simulink model "EspacioDeEstados"  (Simulink 7.9)
settings: Solver=ode45  StartTime=0.0  StopTime=50.0  RelTol=1e-3
undefined symbols (not defined in the file or in its folder): A, B
settings Model: Creator=Paul  LastModifiedBy=Santiago
settings DataIOCC: SignalLoggingSaveFormat=Dataset
settings OptimizationCC: ExpressionDepthLimit=128
settings DebuggingCC: MultiTaskDSMMsg=warning  MultiTaskCondExecSysMsg=none  StrictBusMsg=None
settings RTWCC: IncludeERTFirstTime=on
settings CodeAppCC: CustomSymbolStrType=$N$R$M_T

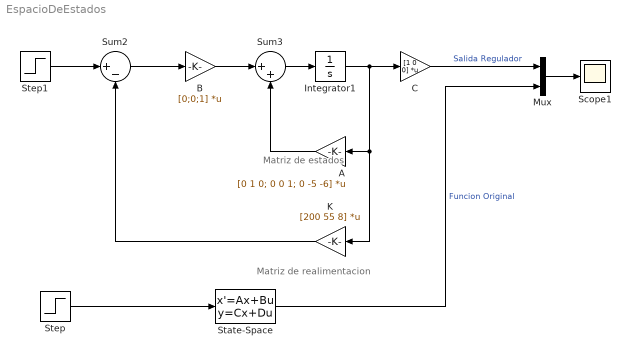
== system EspacioDeEstados ==
  note: Matriz de realimentacion
  note: Matriz de estados
  A : Gain  Gain=[0 1 0; 0 0 1; 0 -5 -6]  Multiplication=Matrix(K*u)
  B : Gain  Gain=[0;0;1]  Multiplication=Matrix(K*u)
  C : Gain  Gain=[1 0 0]  Multiplication=Matrix(K*u)
  Integrator1 : Integrator  InitialCondition=1
  K : Gain  Gain=[200 55 8]  Multiplication=Matrix(K*u)
  Mux : Mux  Inputs=2
  Scope1 : Scope
      settings: ShowLegends=on
  State-Space : StateSpace  A=A  B=B  C=[1 0 0]  D=0  X0=[1 1 1]
  Step : Step  After=0  SampleTime=0
  Step1 : Step  Time=0  After=0  SampleTime=0
  Sum2 : Sum  Inputs=|+-
  Sum3 : Sum  Inputs=|++
  wires:
  Step1/1 -> Sum2/1
  Sum2/1 -> B/1
  B/1 -> Sum3/1
  Sum3/1 -> Integrator1/1
  A/1 -> Sum3/2
  K/1 -> Sum2/2
  Integrator1/1 -> K/1, A/1, C/1
  C/1 -> Mux/1  "Salida Regulador"
  Mux/1 -> Scope1/1
  State-Space/1 -> Mux/2  "Funcion Original"
  Step/1 -> State-Space/1
